simulink model "block_motion_sim"  (R2017a)
settings: Solver=VariableStepAuto  StartTime=0.0  StopTime=tf  MaxStep=.01  RelTol=1e-6
values from neighbouring files (symbols this model uses):
  m = 2    [block_motion_script.m]
  v0 = 1    [block_motion_script.m]
settings Model: Creator=eckelsjd  LastModifiedBy=eckelsjd

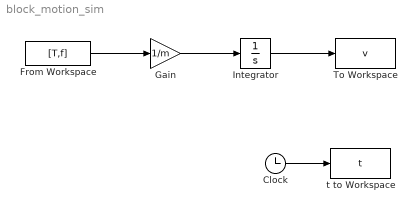
== system block_motion_sim ==
  Clock : Clock
  From Workspace : FromWorkspace  VariableName=[T,f]  SampleTime=0  OutputAfterFinalValue=Setting to zero
  Gain : Gain  Gain=1/m
  Integrator : Integrator  InitialCondition=v0
  To Workspace : ToWorkspace  VariableName=v  SampleTime=-1
  t to Workspace : ToWorkspace  VariableName=t  SampleTime=-1
  wires:
  From Workspace/1 -> Gain/1
  Integrator/1 -> To Workspace/1
  Gain/1 -> Integrator/1
  Clock/1 -> t to Workspace/1
